simulink model "sum1"  (R2025b)
settings: Solver=VariableStepAuto  StartTime=0.0  StopTime=10.0  RelTol=1e-3
values from neighbouring files (symbols this model uses):
  C = double(C)    [ej1.m]

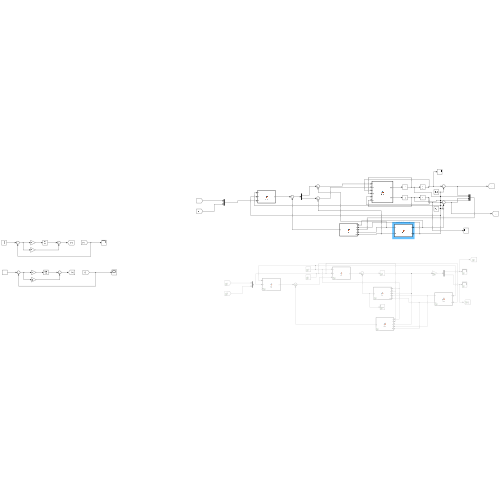
[thumbnail: Simulink's stored preview of the top-level diagram]
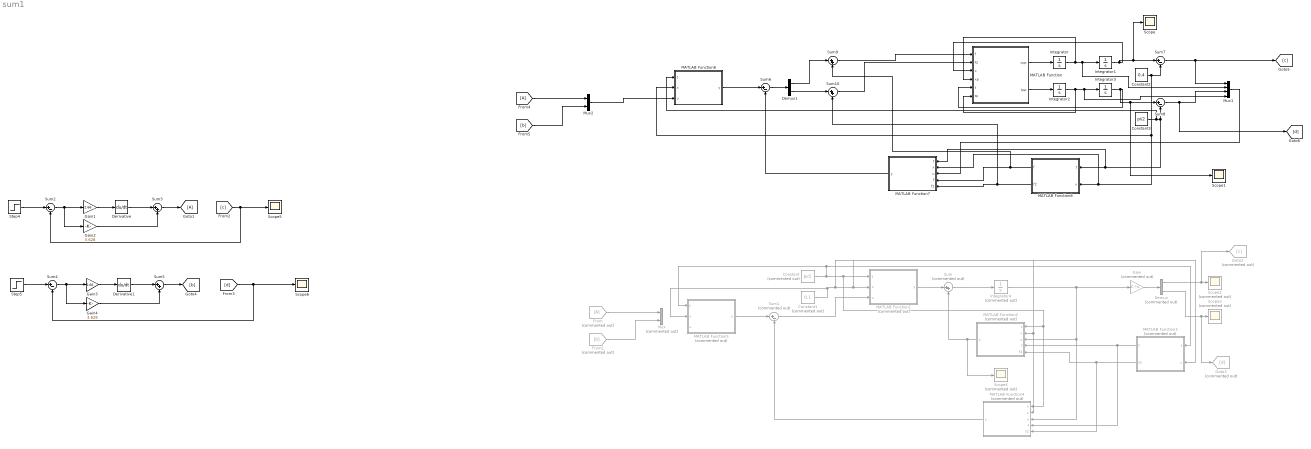
== system sum1 ==
  Constant : Constant  Commented=on  Value=pi/2
  Constant1 : Constant  Commented=on  Value=0.1
  Constant2 : Constant  Value=0.4
  Constant3 : Constant  Value=pi/2
  Demux : Demux  Commented=on  Outputs=2
  Demux1 : Demux  Outputs=2
  Derivative : Derivative
  Derivative1 : Derivative
  From : From  Commented=on
  From1 : From  Commented=on  GotoTag=b
  From4 : From
  Gain : Gain  Commented=on  Gain=C  Multiplication=Matrix(K*u)
  Gain1 : Gain  Gain=2.66
  Gain2 : Gain  Gain=3.628
  Gain3 : Gain  Gain=2.66
  Gain4 : Gain  Gain=3.628
  Goto1 : Goto
  Goto2 : Goto  Commented=on  GotoTag=c
  Goto3 : Goto  Commented=on  GotoTag=d
  Integrator{,1..3} (4 alike) : Integrator
  Integrator4 : Integrator  Commented=on
  MATLAB Function : MATLAB Function  TreatAsAtomicUnit=on
  MATLAB Function1 : MATLAB Function  Commented=on  TreatAsAtomicUnit=on
  MATLAB Function2 : MATLAB Function  Commented=on  TreatAsAtomicUnit=on
  MATLAB Function3 : MATLAB Function  Commented=on  TreatAsAtomicUnit=on
  MATLAB Function4 : MATLAB Function  Commented=on  TreatAsAtomicUnit=on
  MATLAB Function5 : MATLAB Function  Commented=on  TreatAsAtomicUnit=on
  MATLAB Function6 : MATLAB Function  TreatAsAtomicUnit=on
  MATLAB Function7 : MATLAB Function  TreatAsAtomicUnit=on
  MATLAB Function8 : MATLAB Function  TreatAsAtomicUnit=on
  Mux : Mux  Commented=on  Inputs=2
  Mux1 : Mux
  Mux2 : Mux  Inputs=2
  Scope{,1,5..6} (4 alike) : Scope
  Scope2 : Scope  Commented=on
  Scope3 : Scope  Commented=on
  Scope4 : Scope  Commented=on
  Step4 : Step  After=0  SampleTime=0
  Step5 : Step  After=0  SampleTime=0
  Sum : Sum  Commented=on  Inputs=|++
  Sum1 : Sum  Commented=on  Inputs=|+-
  Sum{3,5,9..10} (4 alike) : Sum  Inputs=|++
  Sum{2,4,6..8} (5 alike) : Sum  Inputs=|+-
  wires:
  MATLAB Function/1(xpp) -> Integrator/1
  Integrator/1 -> Mux1/2, Integrator1/1, MATLAB Function/4(xp)
  Integrator1/1 -> Scope/1, Sum7/1, MATLAB Function/3(x)
  MATLAB Function/2(tpp) -> Integrator2/1
  Integrator2/1 -> Mux1/4, Integrator3/1, MATLAB Function/6(tp)
  Integrator3/1 -> Scope1/1, Sum8/1, MATLAB Function/5(t)
  Constant/1 -> MATLAB Function3/1(t), MATLAB Function5/1(t), MATLAB Function4/1(t), MATLAB Function2/1(t), MATLAB Function1/1(t)
  Constant1/1 -> MATLAB Function5/2(x), MATLAB Function3/2(x), MATLAB Function4/2(x), MATLAB Function2/2(x), MATLAB Function1/2(x)
  From/1 -> Mux/1
  From1/1 -> Mux/2
  MATLAB Function1/1(y) -> Sum/1
  Sum/1 -> Integrator4/1
  Integrator4/1 -> MATLAB Function4/3(u), MATLAB Function2/3(u), Gain/1
  Gain/1 -> Demux/1
  Demux/1 -> Goto2/1, Scope2/1
  Demux/2 -> Goto3/1, Scope3/1
  MATLAB Function3/1(f) -> MATLAB Function4/4(f), MATLAB Function2/4(f)
  MATLAB Function3/2(f2) -> MATLAB Function4/5(f2), MATLAB Function2/5(f2)
  MATLAB Function2/1(y) -> Sum/2, Scope4/1
  MATLAB Function4/1(y) -> Sum1/2
  Sum1/1 -> MATLAB Function1/3(u)
  MATLAB Function5/1(y) -> Sum1/1
  Step4/1 -> Sum2/1
  Sum2/1 -> Gain2/1, Gain1/1
  Gain1/1 -> Derivative/1
  Derivative/1 -> Sum3/1
  Gain2/1 -> Sum3/2
  [c] -> Scope5/1, Sum2/2
  Sum3/1 -> Goto1/1
  Sum5/1 -> [b]
  [d] -> Sum4/2, Scope6/1
  Gain4/1 -> Sum5/2
  Derivative1/1 -> Sum5/1
  Gain3/1 -> Derivative1/1
  Sum4/1 -> Gain3/1, Gain4/1
  Step5/1 -> Sum4/1
  MATLAB Function6/1(y) -> Sum6/1
  MATLAB Function7/1(y) -> Sum6/2
  Constant2/1 -> MATLAB Function6/2(x), MATLAB Function7/2(x), MATLAB Function8/2(x), Sum7/2
  Constant3/1 -> MATLAB Function6/1(t), Sum8/2, MATLAB Function7/1(t), MATLAB Function8/1(t)
  MATLAB Function8/1(f) -> Sum9/2, MATLAB Function7/4(f)
  MATLAB Function8/2(f2) -> Sum10/2, MATLAB Function7/5(f2)
  Sum7/1 -> Mux1/1, [c]
  Sum8/1 -> [d], Mux1/3
  Mux1/1 -> MATLAB Function7/3(u)
  Sum6/1 -> Demux1/1
  Demux1/1 -> Sum9/1
  Demux1/2 -> Sum10/1
  Sum9/1 -> MATLAB Function/1(f)
  Sum10/1 -> MATLAB Function/2(f2)
  [b] -> Mux2/2
  From4/1 -> Mux2/1
  Mux2/1 -> MATLAB Function6/3(u)

== matlab function sum1/MATLAB Function1 ==
function y = fcn(t, x, u)
B =[                                          0,                                       0; 1/6 - (25*cos(t)^2)/(6*(25*cos(t)^2 - 150)), -(25*cos(t)*sin(t))/(25*cos(t)^2 - 150);                                          0,                                       0; (50*cos(t))/(25*cos(t)^2 - 150),        (300*sin(t))/(25*cos(t)^2 - 150)]
y=B*u

== matlab function sum1/MATLAB Function ==
function [xpp, tpp] = fcn(f,f2, x, xp, t, tp)
tpp = (25*cos(t)*sin(t)*tp^2 + 2943*sin(t) + 50*f*cos(t) + 300*f2*sin(t) - 5000*x*cos(t))/(25*cos(t)^2 - 150)
xpp = f/6 - (50*x)/3 + (tp^2*sin(t))/12 - (cos(t)*(25*cos(t)*sin(t)*tp^2 + 2943*sin(t) + 50*f*cos(t) + 300*f2*sin(t) - 5000*x*cos(t)))/(12*(25*cos(t)^2 - 150))

== matlab function sum1/MATLAB Function2 ==
function y = fcn(t, x, u, f, f2)
A =[                                         0, 1,                                                                                                                                                                                                                                                                                                    0, 0; (1250*cos(t)^2)/(75*cos(t)^2 - 450) - 50/3, 0, (sin(t)*(2943*sin(t) + 50*f*cos(t) + 300*f2*sin(t) - 5000*x*cos(t)))/(300*cos(t)^2 - 1800) - (cos(t)*(2943*cos(t) + 300*f2*cos(t) - 50*f*sin(t) + 5000*x*sin(t)))/(300*cos(t)^2 - 1800) - (25*cos(t)^2*sin(t)*(2943*sin(t) + 50*f*cos(t) + 300*f2*sin(t) - 5000*x*cos(t)))/(6*(25*cos(t)^2 - 150)^2), 0;                                         0, 0,                                                                                                                                                                                                                                                                                                    0, 1;      -(5000*cos(t))/(25*cos(t)^2 - 150), 0,                                                                                                               (2943*cos(t) + 300*f2*cos(t) - 50*f*sin(t) + 5000*x*sin(t))/(25*cos(t)^2 - 150) + (50*cos(t)*sin(t)*(2943*sin(t) + 50*f*cos(t) + 300*f2*sin(t) - 5000*x*cos(t)))/(25*cos(t)^2 - 150)^2, 0]
 


y=A*u

== matlab function sum1/MATLAB Function3 ==
function [f, f2] = fcn(t, x)
m=1
M=5
g=9.81
l=0.5
k=100
f=k*x
f2=-m*g

== matlab function sum1/MATLAB Function4 ==
function y = fcn(t, x, u, f, f2)
F =[                          (7500*cos(t)^2)/(75*cos(t)^2 - 450) - (2500*cos(t)^2)/(25*cos(t)^2 - 150) - 100, 0,                   (cos(t)*((2943*cos(t) + 300*f2*cos(t) - 50*f*sin(t) + 5000*x*sin(t))/(25*cos(t)^2 - 150) + (50*cos(t)*sin(t)*(2943*sin(t) + 50*f*cos(t) + 300*f2*sin(t) - 5000*x*cos(t)))/(25*cos(t)^2 - 150)^2))/2 - (6*cos(t)*(2943*cos(t) + 300*f2*cos(t) - 50*f*sin(t) + 5000*x*sin(t)))/(300*cos(t)^2 - 1800) + (6*sin(t)*(2943*sin(t) + 50*f*cos(t) + 300*f2*sin(t) - 5000*x*cos(t)))/(300*cos(t)^2 - 1800) - (25*cos(t)^2*sin(t)*(2943*sin(t) + 50*f*cos(t) + 300*f2*sin(t) - 5000*x*cos(t)))/(25*cos(t)^2 - 150)^2, 0;(2500*cos(t))/(sin(t)*(25*cos(t)^2 - 150)) - (cos(t)*((1250*cos(t)^2)/(75*cos(t)^2 - 450) - 50/3))/sin(t), 0, (cos(t)*((cos(t)*(2943*cos(t) + 300*f2*cos(t) - 50*f*sin(t) + 5000*x*sin(t)))/(300*cos(t)^2 - 1800) - (sin(t)*(2943*sin(t) + 50*f*cos(t) + 300*f2*sin(t) - 5000*x*cos(t)))/(300*cos(t)^2 - 1800) + (25*cos(t)^2*sin(t)*(2943*sin(t) + 50*f*cos(t) + 300*f2*sin(t) - 5000*x*cos(t)))/(6*(25*cos(t)^2 - 150)^2)))/sin(t) - ((2943*cos(t) + 300*f2*cos(t) - 50*f*sin(t) + 5000*x*sin(t))/(25*cos(t)^2 - 150) + (50*cos(t)*sin(t)*(2943*sin(t) + 50*f*cos(t) + 300*f2*sin(t) - 5000*x*cos(t)))/(25*cos(t)^2 - 150)^2)/(2*sin(t)), 0]


y=F*u

== matlab function sum1/MATLAB Function5 ==
function y = fcn(t, x, u)
G =[             6,      cos(t)/2; -cos(t)/sin(t), -1/(2*sin(t))]
y=G*u

== matlab function sum1/MATLAB Function6 ==
function y = fcn(t, x, u)
G =[             6,      cos(t)/2; -cos(t)/sin(t), -1/(2*sin(t))]
y=G*u

== matlab function sum1/MATLAB Function7 ==
function y = fcn(t, x, u, f, f2)
F =[                          (7500*cos(t)^2)/(75*cos(t)^2 - 450) - (2500*cos(t)^2)/(25*cos(t)^2 - 150) - 100, 0,                   (cos(t)*((2943*cos(t) + 300*f2*cos(t) - 50*f*sin(t) + 5000*x*sin(t))/(25*cos(t)^2 - 150) + (50*cos(t)*sin(t)*(2943*sin(t) + 50*f*cos(t) + 300*f2*sin(t) - 5000*x*cos(t)))/(25*cos(t)^2 - 150)^2))/2 - (6*cos(t)*(2943*cos(t) + 300*f2*cos(t) - 50*f*sin(t) + 5000*x*sin(t)))/(300*cos(t)^2 - 1800) + (6*sin(t)*(2943*sin(t) + 50*f*cos(t) + 300*f2*sin(t) - 5000*x*cos(t)))/(300*cos(t)^2 - 1800) - (25*cos(t)^2*sin(t)*(2943*sin(t) + 50*f*cos(t) + 300*f2*sin(t) - 5000*x*cos(t)))/(25*cos(t)^2 - 150)^2, 0;(2500*cos(t))/(sin(t)*(25*cos(t)^2 - 150)) - (cos(t)*((1250*cos(t)^2)/(75*cos(t)^2 - 450) - 50/3))/sin(t), 0, (cos(t)*((cos(t)*(2943*cos(t) + 300*f2*cos(t) - 50*f*sin(t) + 5000*x*sin(t)))/(300*cos(t)^2 - 1800) - (sin(t)*(2943*sin(t) + 50*f*cos(t) + 300*f2*sin(t) - 5000*x*cos(t)))/(300*cos(t)^2 - 1800) + (25*cos(t)^2*sin(t)*(2943*sin(t) + 50*f*cos(t) + 300*f2*sin(t) - 5000*x*cos(t)))/(6*(25*cos(t)^2 - 150)^2)))/sin(t) - ((2943*cos(t) + 300*f2*cos(t) - 50*f*sin(t) + 5000*x*sin(t))/(25*cos(t)^2 - 150) + (50*cos(t)*sin(t)*(2943*sin(t) + 50*f*cos(t) + 300*f2*sin(t) - 5000*x*cos(t)))/(25*cos(t)^2 - 150)^2)/(2*sin(t)), 0]


y=F*u

== matlab function sum1/MATLAB Function8 ==
function [f, f2] = fcn(t, x)
m=1
M=5
g=9.81
l=0.5
k=100
f=k*x
f2=-m*g
